simulink subsystem "Find_Target_Pose"  (R2023b)
settings: Solver=VariableStepAuto  StartTime=0.0  StopTime=10.0  RelTol=1e-3
undefined symbols (not defined in the file): Spline_Max_Num_RefPoses
libraries: simulink x2
settings Model: Creator=FIRSTMentor  LastModifiedBy=ander

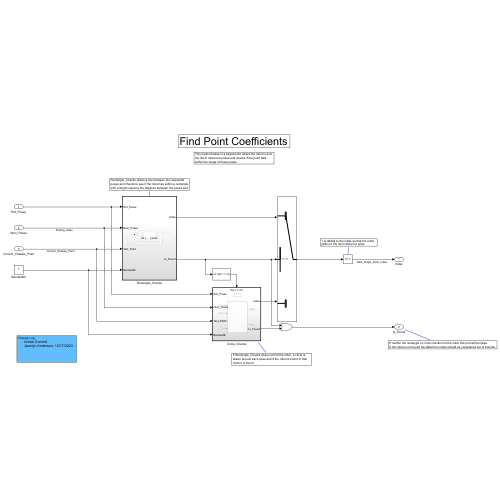
[thumbnail: Simulink's stored preview of the top-level diagram]
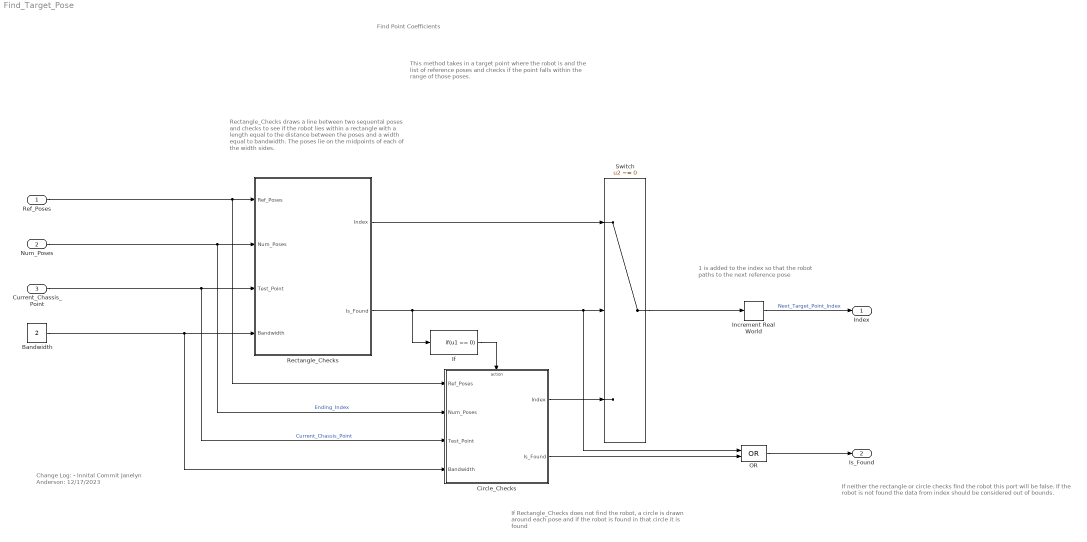
== system Find_Target_Pose ==
  note: 1 is added to the index so that the robot paths to the next reference pose
  note: If neither the rectangle or circle checks find the robot this port will be false.
      | If the robot is not found the data from index should be considered out of bounds.
  note: Change Log:
      | - Innital Commit
      | Janelyn Anderson: 12/17/2023
  note: Find Point Coefficients
  note: This method takes in a target point where the robot is and the list of reference poses and checks if the point falls within the range of those poses.
  note: Rectangle_Checks draws a line between two sequental poses and checks to see if the robot lies within a rectangle with a length equal to the distance between the poses and a width equal to bandwidth. The poses lie on the midpoints of each of the width sides.
  note: If Rectangle_Checks does not find the robot, a circle is drawn around each pose and if the robot is found in that circle it is found
  Ref_Poses : Inport  OutDataTypeStr=double  PortDimensions=[Spline_Max_Num_RefPoses 2]
  Num_Poses : Inport  Port=2  Unit=1  PortDimensions=1
  Current_Chassis_Point : Inport  Port=3  OutDataTypeStr=double  Unit=m  PortDimensions=[1 2]
  Bandwidth : Constant  Value=2
  Circle_Checks : Subsystem  TreatAsAtomicUnit=on
  If : If  IfExpression=u1 == 0  ShowElse=off
  Increment Real World : simulink/Additional Math & Discrete/Additional Math: Increment - Decrement/Increment Real World
  OR : Logic  Operator=OR  AllPortsSameDT=off  OutDataTypeStr=boolean
  Rectangle_Checks : Subsystem  TreatAsAtomicUnit=on
  Switch : Switch  Criteria=u2 ~= 0  SaturateOnIntegerOverflow=off  InputSameDT=off
  Index : Outport
  Is_Found : Outport  Port=2
  wires:
  Num_Poses/1 -> Rectangle_Checks/2(Num_Poses), Circle_Checks/2(Num_Poses)  "Ending_Index"
  Rectangle_Checks/1(Index) -> Switch/1
  Current_Chassis_Point/1 -> Rectangle_Checks/3(Test_Point), Circle_Checks/3(Test_Point)  "Current_Chassis_Point"
  If/1 -> Circle_Checks/Action
  Rectangle_Checks/2(Is_Found) -> If/1, Switch/2, OR/1
  Switch/1 -> Increment Real World/1
  Ref_Poses/1 -> Rectangle_Checks/1(Ref_Poses), Circle_Checks/1(Ref_Poses)
  Increment Real World/1 -> Index/1  "Next_Target_Point_Index"
  OR/1 -> Is_Found/1
  Circle_Checks/1(Index) -> Switch/3
  Bandwidth/1 -> Rectangle_Checks/4(Bandwidth), Circle_Checks/4(Bandwidth)
  Circle_Checks/2(Is_Found) -> OR/2

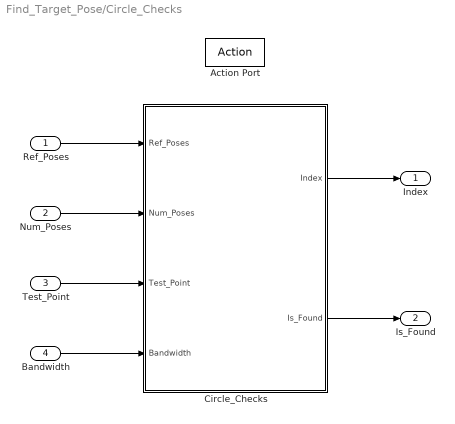
== system Find_Target_Pose/Circle_Checks ==
  Ref_Poses : Inport
  Num_Poses : Inport  Port=2
  Test_Point : Inport  Port=3
  Bandwidth : Inport  Port=4
  Action Port : ActionPort
  Circle_Checks : Subsystem  TreatAsAtomicUnit=on
  Index : Outport
  Is_Found : Outport  Port=2
  wires:
  Ref_Poses/1 -> Circle_Checks/1(Ref_Poses)
  Test_Point/1 -> Circle_Checks/3(Test_Point)
  Bandwidth/1 -> Circle_Checks/4(Bandwidth)
  Circle_Checks/1(Index) -> Index/1
  Num_Poses/1 -> Circle_Checks/2(Num_Poses)
  Circle_Checks/2(Is_Found) -> Is_Found/1

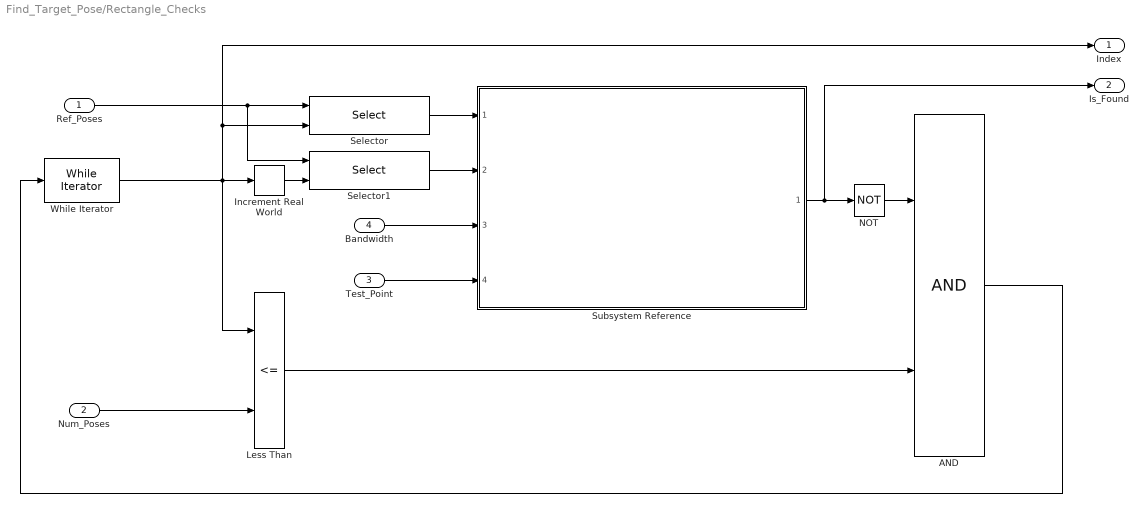
== system Find_Target_Pose/Rectangle_Checks ==
  Ref_Poses : Inport
  Num_Poses : Inport  Port=2
  Test_Point : Inport  Port=3
  Bandwidth : Inport  Port=4
  AND : Logic  AllPortsSameDT=off  OutDataTypeStr=boolean
  Increment Real World : simulink/Additional Math & Discrete/Additional Math: Increment - Decrement/Increment Real World
  Less Than : RelationalOperator  Operator=<=  OutDataTypeStr=boolean  RndMeth=Simplest  InputSameDT=off
  NOT : Logic  Operator=NOT  AllPortsSameDT=off  OutDataTypeStr=boolean
  Selector : Selector  NumberOfDimensions=2  InputPortWidth=3  IndexOptions=Index vector (port),Select all  Indices=[1 3],1  OutputSizes=1,1
  Selector1 : Selector  NumberOfDimensions=2  InputPortWidth=3  IndexOptions=Index vector (port),Select all  Indices=[1 3],1  OutputSizes=1,1
  Subsystem Reference : Subsystem  ReferencedSubsystem=Bandwidth_Check_Between_Two_Points
  While Iterator : WhileIterator  MaxIters=Spline_Max_Num_RefPoses-1  WhileBlockType=do-while  ShowIterationPort=on
  Index : Outport
  Is_Found : Outport  Port=2
  wires:
  Test_Point/1 -> Subsystem Reference/4
  Bandwidth/1 -> Subsystem Reference/3
  Selector/1 -> Subsystem Reference/1
  Selector1/1 -> Subsystem Reference/2
  Ref_Poses/1 -> Selector1/1, Selector/1
  NOT/1 -> AND/1
  Increment Real World/1 -> Selector1/2
  While Iterator/1 -> Less Than/1, Increment Real World/1, Index/1, Selector/2
  Subsystem Reference/1 -> Is_Found/1, NOT/1
  Less Than/1 -> AND/2
  AND/1 -> While Iterator/1
  Num_Poses/1 -> Less Than/2

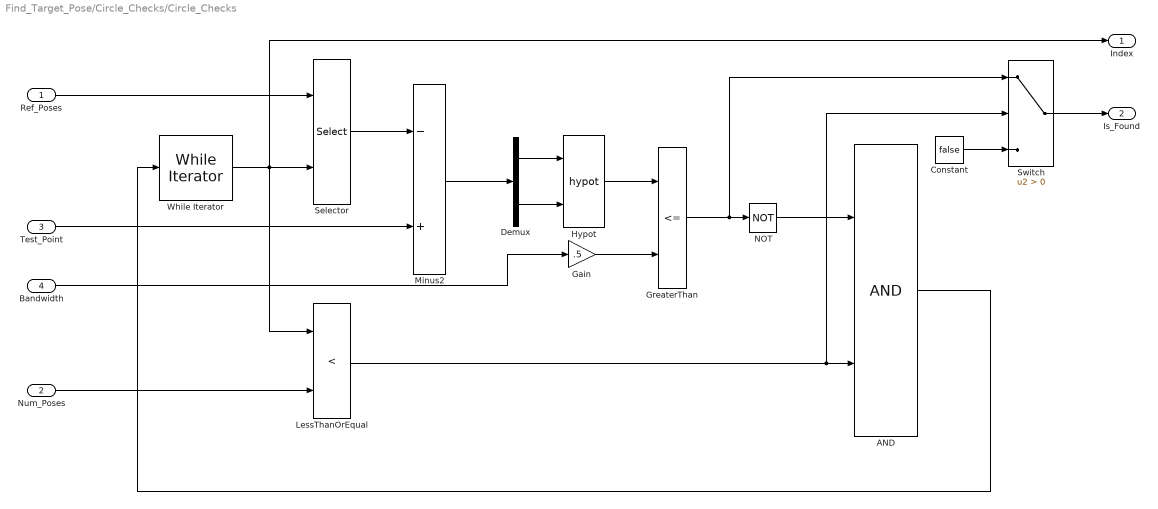
== system Find_Target_Pose/Circle_Checks/Circle_Checks ==
  Ref_Poses : Inport
  Num_Poses : Inport  Port=2
  Test_Point : Inport  Port=3
  Bandwidth : Inport  Port=4
  AND : Logic  AllPortsSameDT=off  OutDataTypeStr=boolean
  Constant : Constant  Value=false
  Demux : Demux  Outputs=2
  Gain : Gain  Gain=.5
  GreaterThan : RelationalOperator  Operator=<=  OutDataTypeStr=boolean  RndMeth=Simplest  InputSameDT=off
  Hypot : Math  Operator=hypot
  LessThanOrEqual : RelationalOperator  Operator=<  OutDataTypeStr=boolean  RndMeth=Simplest  InputSameDT=off
  Minus2 : Sum  Inputs=-+
  NOT : Logic  Operator=NOT  AllPortsSameDT=off  OutDataTypeStr=boolean
  Selector : Selector  NumberOfDimensions=2  InputPortWidth=3  IndexOptions=Index vector (port),Select all  Indices=[1 3],1  OutputSizes=1,1
  Switch : Switch  Criteria=u2 > Threshold  SaturateOnIntegerOverflow=off  InputSameDT=off
  While Iterator : WhileIterator  MaxIters=Spline_Max_Num_RefPoses  WhileBlockType=do-while  ShowIterationPort=on
  Index : Outport
  Is_Found : Outport  Port=2
  wires:
  Demux/1 -> Hypot/1
  Num_Poses/1 -> LessThanOrEqual/2
  LessThanOrEqual/1 -> Switch/2, AND/2
  Selector/1 -> Minus2/1
  Ref_Poses/1 -> Selector/1
  Test_Point/1 -> Minus2/2
  Minus2/1 -> Demux/1
  Demux/2 -> Hypot/2
  Bandwidth/1 -> Gain/1
  Hypot/1 -> GreaterThan/1
  Gain/1 -> GreaterThan/2
  GreaterThan/1 -> Switch/1, NOT/1
  AND/1 -> While Iterator/1
  While Iterator/1 -> LessThanOrEqual/1, Selector/2, Index/1
  NOT/1 -> AND/1
  Switch/1 -> Is_Found/1
  Constant/1 -> Switch/3
